simulink model "cmult_core"  (R2013a)
settings: Solver=ode45  StartTime=0.0  StopTime=10.0  RelTol=1e-3
libraries: xbsIndex_r4 x2035, casper_library_misc x116, casper_library_multipliers x36
(part 3 of 23)

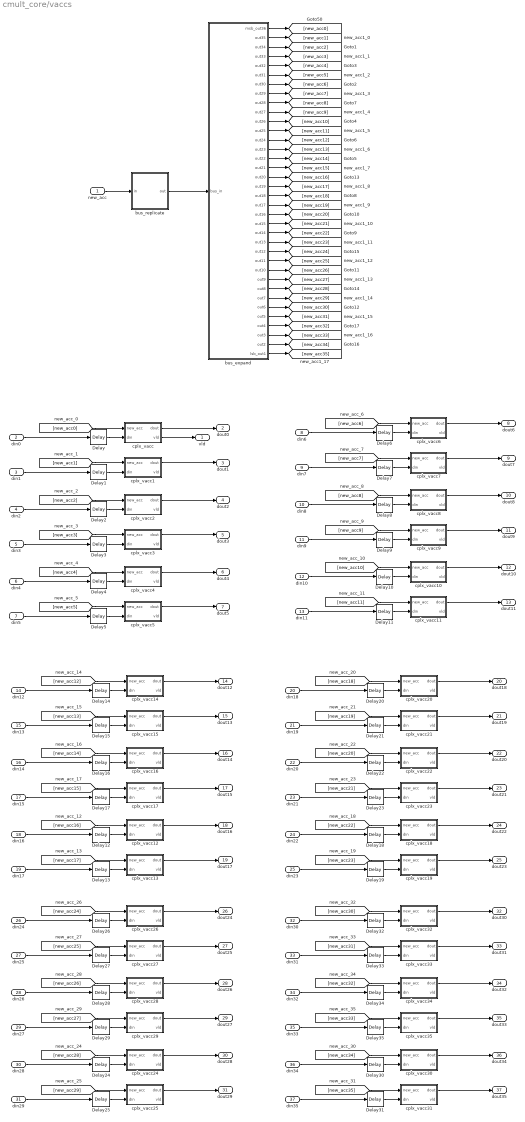
== system cmult_core/vaccs ==
  new_acc : Inport
  din0 : Inport  Port=2
  din1 : Inport  Port=3
  din2 : Inport  Port=4
  din3 : Inport  Port=5
  din4 : Inport  Port=6
  din5 : Inport  Port=7
  din6 : Inport  Port=8
  din7 : Inport  Port=9
  din8 : Inport  Port=10
  din9 : Inport  Port=11
  din10 : Inport  Port=12
  din11 : Inport  Port=13
  din12 : Inport  Port=14
  din13 : Inport  Port=15
  din14 : Inport  Port=16
  din15 : Inport  Port=17
  din16 : Inport  Port=18
  din17 : Inport  Port=19
  din18 : Inport  Port=20
  din19 : Inport  Port=21
  din20 : Inport  Port=22
  din21 : Inport  Port=23
  din22 : Inport  Port=24
  din23 : Inport  Port=25
  din24 : Inport  Port=26
  din25 : Inport  Port=27
  din26 : Inport  Port=28
  din27 : Inport  Port=29
  din28 : Inport  Port=30
  din29 : Inport  Port=31
  din30 : Inport  Port=32
  din31 : Inport  Port=33
  din32 : Inport  Port=34
  din33 : Inport  Port=35
  din34 : Inport  Port=36
  din35 : Inport  Port=37
  Delay{,1..35} (36 alike) : xbsIndex_r4/Delay  rst=off  infoeditControl=Selection of Reset will increase slice count due to use of real FFs and instead of SRLs  en=off  latency=5  dbl_ovrd=off  reg_retiming=on  block_type=delay
  bus_expand : Subsystem  AncestorBlock=casper_library_flow_control/bus_expand  mask(bus_expand){mode=divisions of equal size, outputNum=36, outputWidth=1, outputBinaryPt=0, outputArithmeticType=2, show_format=off, outputToWorkspace=off, variablePrefix=out, outputToModelAsWell=on}
      mask prompts: outputNum "Number of outputs:"; outputWidth "Output width:"; outputBinaryPt "Output binary point position:"; outputArithmeticType "Output arithmetic type (ufix=0, fix=1, bool=2):"; show_format "Print format string?"; outputToWorkspace "Output to workspace?"; variablePrefix "Variable name prefix:"; outputToModelAsWell "Output to model as well?"
      mask help:
      | Expands a 'bus' made using a bus_create or Xilinx
      | concat block.
      | The input will be divided into the specified number
      | of outputs with the specified arithmetic types.
      | Divisions are made from most significant bit.
      mask init: same as cmult_core/cross_multiplier/unpack0
      settings: AttributesFormatString=36 outputs
      mask TypeOptions mode: divisions of equal size | divisions of arbitrary size
      mask Callback mode: bus_expand_callback();
      mask Callback outputWidth: bus_expand_callback();
      mask Callback outputToWorkspace: bus_expand_callback();
  bus_replicate : Subsystem  AncestorBlock=casper_library_bus/bus_replicate  mask(bus_replicate){replication=36, latency=5, misc=off, implementation=core}
      mask prompts: replication "replication factor"; misc "misc support"; implementation "delay implementation"
      mask help: Output bus formed by replicating input bus a number of times
      mask init:
      | bus_replicate_init(gcb, ...
      |     'replication', replication, ...
      |     'latency', latency, ...
      |     'implementation', implementation, ...
      |     'misc', misc);
      mask TypeOptions implementation: core | behavioral
  cplx_vacc : Subsystem  mask{vacc_len=vacc_len}
      mask prompts: vacc_len "vector length"
  cplx_vacc1 : Subsystem  mask{vacc_len=vacc_len}
      mask prompts: vacc_len "vector length"
  cplx_vacc10 : Subsystem  mask{vacc_len=vacc_len}
      mask prompts: vacc_len "vector length"
  cplx_vacc11 : Subsystem  mask{vacc_len=vacc_len}
      mask prompts: vacc_len "vector length"
  cplx_vacc12 : Subsystem  mask{vacc_len=vacc_len}
      mask prompts: vacc_len "vector length"
  cplx_vacc13 : Subsystem  mask{vacc_len=vacc_len}
      mask prompts: vacc_len "vector length"
  cplx_vacc14 : Subsystem  mask{vacc_len=vacc_len}
      mask prompts: vacc_len "vector length"
  cplx_vacc15 : Subsystem  mask{vacc_len=vacc_len}
      mask prompts: vacc_len "vector length"
  cplx_vacc16 : Subsystem  mask{vacc_len=vacc_len}
      mask prompts: vacc_len "vector length"
  cplx_vacc17 : Subsystem  mask{vacc_len=vacc_len}
      mask prompts: vacc_len "vector length"
  cplx_vacc18 : Subsystem  mask{vacc_len=vacc_len}
      mask prompts: vacc_len "vector length"
  cplx_vacc19 : Subsystem  mask{vacc_len=vacc_len}
      mask prompts: vacc_len "vector length"
  cplx_vacc2 : Subsystem  mask{vacc_len=vacc_len}
      mask prompts: vacc_len "vector length"
  cplx_vacc20 : Subsystem  mask{vacc_len=vacc_len}
      mask prompts: vacc_len "vector length"
  cplx_vacc21 : Subsystem  mask{vacc_len=vacc_len}
      mask prompts: vacc_len "vector length"
  cplx_vacc22 : Subsystem  mask{vacc_len=vacc_len}
      mask prompts: vacc_len "vector length"
  cplx_vacc23 : Subsystem  mask{vacc_len=vacc_len}
      mask prompts: vacc_len "vector length"
  cplx_vacc24 : Subsystem  mask{vacc_len=vacc_len}
      mask prompts: vacc_len "vector length"
  cplx_vacc25 : Subsystem  mask{vacc_len=vacc_len}
      mask prompts: vacc_len "vector length"
  cplx_vacc26 : Subsystem  mask{vacc_len=vacc_len}
      mask prompts: vacc_len "vector length"
  cplx_vacc27 : Subsystem  mask{vacc_len=vacc_len}
      mask prompts: vacc_len "vector length"
  cplx_vacc28 : Subsystem  mask{vacc_len=vacc_len}
      mask prompts: vacc_len "vector length"
  cplx_vacc29 : Subsystem  mask{vacc_len=vacc_len}
      mask prompts: vacc_len "vector length"
  cplx_vacc3 : Subsystem  mask{vacc_len=vacc_len}
      mask prompts: vacc_len "vector length"
  cplx_vacc30 : Subsystem  mask{vacc_len=vacc_len}
      mask prompts: vacc_len "vector length"
  cplx_vacc31 : Subsystem  mask{vacc_len=vacc_len}
      mask prompts: vacc_len "vector length"
  cplx_vacc32 : Subsystem  mask{vacc_len=vacc_len}
      mask prompts: vacc_len "vector length"
  cplx_vacc33 : Subsystem  mask{vacc_len=vacc_len}
      mask prompts: vacc_len "vector length"
  cplx_vacc34 : Subsystem  mask{vacc_len=vacc_len}
      mask prompts: vacc_len "vector length"
  cplx_vacc35 : Subsystem  mask{vacc_len=vacc_len}
      mask prompts: vacc_len "vector length"
  cplx_vacc4 : Subsystem  mask{vacc_len=vacc_len}
      mask prompts: vacc_len "vector length"
  cplx_vacc5 : Subsystem  mask{vacc_len=vacc_len}
      mask prompts: vacc_len "vector length"
  cplx_vacc6 : Subsystem  mask{vacc_len=vacc_len}
      mask prompts: vacc_len "vector length"
  cplx_vacc7 : Subsystem  mask{vacc_len=vacc_len}
      mask prompts: vacc_len "vector length"
  cplx_vacc8 : Subsystem  mask{vacc_len=vacc_len}
      mask prompts: vacc_len "vector length"
  cplx_vacc9 : Subsystem  mask{vacc_len=vacc_len}
      mask prompts: vacc_len "vector length"
  vld : Outport
  dout0 : Outport  Port=2
  dout1 : Outport  Port=3
  dout2 : Outport  Port=4
  dout3 : Outport  Port=5
  dout4 : Outport  Port=6
  dout5 : Outport  Port=7
  dout6 : Outport  Port=8
  dout7 : Outport  Port=9
  dout8 : Outport  Port=10
  dout9 : Outport  Port=11
  dout10 : Outport  Port=12
  dout11 : Outport  Port=13
  dout12 : Outport  Port=14
  dout13 : Outport  Port=15
  dout14 : Outport  Port=16
  dout15 : Outport  Port=17
  dout16 : Outport  Port=18
  dout17 : Outport  Port=19
  dout18 : Outport  Port=20
  dout19 : Outport  Port=21
  dout20 : Outport  Port=22
  dout21 : Outport  Port=23
  dout22 : Outport  Port=24
  dout23 : Outport  Port=25
  dout24 : Outport  Port=26
  dout25 : Outport  Port=27
  dout26 : Outport  Port=28
  dout27 : Outport  Port=29
  dout28 : Outport  Port=30
  dout29 : Outport  Port=31
  dout30 : Outport  Port=32
  dout31 : Outport  Port=33
  dout32 : Outport  Port=34
  dout33 : Outport  Port=35
  dout34 : Outport  Port=36
  dout35 : Outport  Port=37
  wires:
  cplx_vacc/1(dout) -> dout0/1
  cplx_vacc/2(vld) -> vld/1
  din0/1 -> Delay/1
  [new_acc0] -> cplx_vacc/1(new_acc)
  new_acc/1 -> bus_replicate/1(in)
  bus_replicate/1(out) -> bus_expand/1(bus_in)
  bus_expand/28(out9) -> [new_acc27]
  bus_expand/36(lsb_out1) -> [new_acc35]
  bus_expand/35(out2) -> [new_acc34]
  bus_expand/30(out7) -> [new_acc29]
  bus_expand/23(out14) -> [new_acc22]
  bus_expand/24(out13) -> [new_acc23]
  bus_expand/32(out5) -> [new_acc31]
  bus_expand/11(out26) -> [new_acc10]
  bus_expand/31(out6) -> [new_acc30]
  bus_expand/15(out22) -> [new_acc14]
  bus_expand/8(out29) -> [new_acc7]
  bus_expand/26(out11) -> [new_acc25]
  bus_expand/33(out4) -> [new_acc32]
  bus_expand/22(out15) -> [new_acc21]
  bus_expand/34(out3) -> [new_acc33]
  bus_expand/27(out10) -> [new_acc26]
  bus_expand/9(out28) -> [new_acc8]
  bus_expand/18(out19) -> [new_acc17]
  bus_expand/6(out31) -> [new_acc5]
  bus_expand/10(out27) -> [new_acc9]
  bus_expand/13(out24) -> [new_acc12]
  bus_expand/25(out12) -> [new_acc24]
  bus_expand/14(out23) -> [new_acc13]
  bus_expand/20(out17) -> [new_acc19]
  bus_expand/19(out18) -> [new_acc18]
  bus_expand/3(out34) -> [new_acc2]
  bus_expand/29(out8) -> [new_acc28]
  bus_expand/7(out30) -> [new_acc6]
  bus_expand/16(out21) -> [new_acc15]
  bus_expand/4(out33) -> [new_acc3]
  bus_expand/1(msb_out36) -> [new_acc0]
  bus_expand/2(out35) -> [new_acc1]
  bus_expand/17(out20) -> [new_acc16]
  bus_expand/21(out16) -> [new_acc20]
  bus_expand/12(out25) -> [new_acc11]
  bus_expand/5(out32) -> [new_acc4]
  Delay/1 -> cplx_vacc/2(din)
  cplx_vacc1/1(dout) -> dout1/1
  din1/1 -> Delay1/1
  [new_acc1] -> cplx_vacc1/1(new_acc)
  Delay1/1 -> cplx_vacc1/2(din)
  cplx_vacc2/1(dout) -> dout2/1
  din2/1 -> Delay2/1
  [new_acc2] -> cplx_vacc2/1(new_acc)
  Delay2/1 -> cplx_vacc2/2(din)
  cplx_vacc3/1(dout) -> dout3/1
  din3/1 -> Delay3/1
  [new_acc3] -> cplx_vacc3/1(new_acc)
  Delay3/1 -> cplx_vacc3/2(din)
  cplx_vacc4/1(dout) -> dout4/1
  din4/1 -> Delay4/1
  [new_acc4] -> cplx_vacc4/1(new_acc)
  Delay4/1 -> cplx_vacc4/2(din)
  cplx_vacc5/1(dout) -> dout5/1
  din5/1 -> Delay5/1
  [new_acc5] -> cplx_vacc5/1(new_acc)
  Delay5/1 -> cplx_vacc5/2(din)
  cplx_vacc6/1(dout) -> dout6/1
  din6/1 -> Delay6/1
  [new_acc6] -> cplx_vacc6/1(new_acc)
  Delay6/1 -> cplx_vacc6/2(din)
  cplx_vacc7/1(dout) -> dout7/1
  din7/1 -> Delay7/1
  [new_acc7] -> cplx_vacc7/1(new_acc)
  Delay7/1 -> cplx_vacc7/2(din)
  cplx_vacc8/1(dout) -> dout8/1
  din8/1 -> Delay8/1
  [new_acc8] -> cplx_vacc8/1(new_acc)
  Delay8/1 -> cplx_vacc8/2(din)
  cplx_vacc9/1(dout) -> dout9/1
  din9/1 -> Delay9/1
  [new_acc9] -> cplx_vacc9/1(new_acc)
  Delay9/1 -> cplx_vacc9/2(din)
  cplx_vacc10/1(dout) -> dout10/1
  din10/1 -> Delay10/1
  [new_acc10] -> cplx_vacc10/1(new_acc)
  Delay10/1 -> cplx_vacc10/2(din)
  cplx_vacc11/1(dout) -> dout11/1
  din11/1 -> Delay11/1
  [new_acc11] -> cplx_vacc11/1(new_acc)
  Delay11/1 -> cplx_vacc11/2(din)
  cplx_vacc14/1(dout) -> dout12/1
  din12/1 -> Delay14/1
  [new_acc12] -> cplx_vacc14/1(new_acc)
  Delay14/1 -> cplx_vacc14/2(din)
  cplx_vacc15/1(dout) -> dout13/1
  din13/1 -> Delay15/1
  [new_acc13] -> cplx_vacc15/1(new_acc)
  Delay15/1 -> cplx_vacc15/2(din)
  cplx_vacc16/1(dout) -> dout14/1
  din14/1 -> Delay16/1
  [new_acc14] -> cplx_vacc16/1(new_acc)
  Delay16/1 -> cplx_vacc16/2(din)
  cplx_vacc17/1(dout) -> dout15/1
  din15/1 -> Delay17/1
  [new_acc15] -> cplx_vacc17/1(new_acc)
  Delay17/1 -> cplx_vacc17/2(din)
  cplx_vacc12/1(dout) -> dout16/1
  din16/1 -> Delay12/1
  [new_acc16] -> cplx_vacc12/1(new_acc)
  Delay12/1 -> cplx_vacc12/2(din)
  cplx_vacc13/1(dout) -> dout17/1
  din17/1 -> Delay13/1
  [new_acc17] -> cplx_vacc13/1(new_acc)
  Delay13/1 -> cplx_vacc13/2(din)
  cplx_vacc20/1(dout) -> dout18/1
  din18/1 -> Delay20/1
  [new_acc18] -> cplx_vacc20/1(new_acc)
  Delay20/1 -> cplx_vacc20/2(din)
  cplx_vacc21/1(dout) -> dout19/1
  din19/1 -> Delay21/1
  [new_acc19] -> cplx_vacc21/1(new_acc)
  Delay21/1 -> cplx_vacc21/2(din)
  cplx_vacc22/1(dout) -> dout20/1
  din20/1 -> Delay22/1
  [new_acc20] -> cplx_vacc22/1(new_acc)
  Delay22/1 -> cplx_vacc22/2(din)
  cplx_vacc23/1(dout) -> dout21/1
  din21/1 -> Delay23/1
  [new_acc21] -> cplx_vacc23/1(new_acc)
  Delay23/1 -> cplx_vacc23/2(din)
  cplx_vacc18/1(dout) -> dout22/1
  din22/1 -> Delay18/1
  [new_acc22] -> cplx_vacc18/1(new_acc)
  Delay18/1 -> cplx_vacc18/2(din)
  cplx_vacc19/1(dout) -> dout23/1
  din23/1 -> Delay19/1
  [new_acc23] -> cplx_vacc19/1(new_acc)
  Delay19/1 -> cplx_vacc19/2(din)
  cplx_vacc26/1(dout) -> dout24/1
  din24/1 -> Delay26/1
  [new_acc24] -> cplx_vacc26/1(new_acc)
  Delay26/1 -> cplx_vacc26/2(din)
  cplx_vacc27/1(dout) -> dout25/1
  din25/1 -> Delay27/1
  [new_acc25] -> cplx_vacc27/1(new_acc)
  Delay27/1 -> cplx_vacc27/2(din)
  cplx_vacc28/1(dout) -> dout26/1
  din26/1 -> Delay28/1
  [new_acc26] -> cplx_vacc28/1(new_acc)
  Delay28/1 -> cplx_vacc28/2(din)
  cplx_vacc29/1(dout) -> dout27/1
  din27/1 -> Delay29/1
  [new_acc27] -> cplx_vacc29/1(new_acc)
  Delay29/1 -> cplx_vacc29/2(din)
  cplx_vacc24/1(dout) -> dout28/1
  din28/1 -> Delay24/1
  [new_acc28] -> cplx_vacc24/1(new_acc)
  Delay24/1 -> cplx_vacc24/2(din)
  cplx_vacc25/1(dout) -> dout29/1
  din29/1 -> Delay25/1
  [new_acc29] -> cplx_vacc25/1(new_acc)
  Delay25/1 -> cplx_vacc25/2(din)
  cplx_vacc32/1(dout) -> dout30/1
  din30/1 -> Delay32/1
  [new_acc30] -> cplx_vacc32/1(new_acc)
  Delay32/1 -> cplx_vacc32/2(din)
  cplx_vacc33/1(dout) -> dout31/1
  din31/1 -> Delay33/1
  [new_acc31] -> cplx_vacc33/1(new_acc)
  Delay33/1 -> cplx_vacc33/2(din)
  cplx_vacc34/1(dout) -> dout32/1
  din32/1 -> Delay34/1
  [new_acc32] -> cplx_vacc34/1(new_acc)
  Delay34/1 -> cplx_vacc34/2(din)
  cplx_vacc35/1(dout) -> dout33/1
  din33/1 -> Delay35/1
  [new_acc33] -> cplx_vacc35/1(new_acc)
  Delay35/1 -> cplx_vacc35/2(din)
  cplx_vacc30/1(dout) -> dout34/1
  din34/1 -> Delay30/1
  [new_acc34] -> cplx_vacc30/1(new_acc)
  Delay30/1 -> cplx_vacc30/2(din)
  cplx_vacc31/1(dout) -> dout35/1
  din35/1 -> Delay31/1
  [new_acc35] -> cplx_vacc31/1(new_acc)
  Delay31/1 -> cplx_vacc31/2(din)

== system cmult_core/cross_multiplier/cvrt0_0_0_imag ==
  din : Inport
  convert : Subsystem  AncestorBlock=casper_library_misc/convert  mask(convert){bin_pt_in=binary_point_i, n_bits_out=bit_width_o, bin_pt_out=binary_point_o, quantization=Truncate, overflow=Wrap, latency=latency, adder_imp=Fabric}
      mask prompts: bin_pt_in "Binary Point In"; n_bits_out "Bit Width Out"; bin_pt_out "Binary Point Out"; adder_imp "Adder Implementation"
      mask help:
      | Convert input value to the specified bit width and precision.
      |
      | Does not support upscaling number of fractional bits (eg 8_5 to 8_4 is ok, but not 8_4 to 8_5).
      mask init:
      | convert_init(gcb, ...
      |     'bin_pt_in',bin_pt_in, ...
      |     'n_bits_out',n_bits_out,...
      |     'bin_pt_out',bin_pt_out, ...
      |     'quantization',quantization,...
      |     'overflow',overflow,...
      |     'latency',latency,...
      |     'adder_imp',adder_imp);
      settings: AttributesFormatString=|
      | N_14 ==> 17_14
      | truncate, wrap
      | latency = 0
      mask Help:
      | <pre>
      | Description::
      | 
      | Outputs converted version of the input.
      | 
      | Mask Parameters::
      | 
      | Binary Point In (bin_pt_in): Specifies the binary point location in the input.
      | 
      | Bit Width Out (n_bits_out): Specifies the width of the output.
      | 
      | Binary Point Out (bin_pt_out): Specifies the binary point location in the output.
      | 
      | Quantization (quantization): Specifies quantization handling.
      | 
      | Overflow (overflow): Specifies overflow handling.
      | 
      | Latency (latency): Specifies the latency of the underlying adder block, which is the overall
      | latency of this block as well.
      | Adder Implementation (adder_imp) specifies whether the adder should be implemented in DSP or logic. In either case, pipelining is enabled.</pre>
      mask TypeOptions quantization: Truncate | Round  (unbiased: +/- Inf) | Round  (unbiased: Even Values) | Round  (unbiased: Zero) | Round  (unbiased: Odd Values) | Round  (biased: Up) | Round  (biased: Down)
      mask TypeOptions overflow: Wrap | Saturate | Error
      mask TypeOptions adder_imp: Fabric | DSP48 | Behavioural
  never : xbsIndex_r4/Constant  const=0  gui_display_data_type=Fixed-point  arith_type=Boolean  n_bits=16  bin_pt=14  preci_type=Single  exp_width=8  frac_width=24  explicit_period=on  period=1  equ=P=C  opselect=C  inp2=PCIN>>17  opr=+  inp1=P  carry=CIN  dbl_ovrd=off  block_type=constant
  dout : Outport
  of : Outport  Port=2
  wires:
  din/1 -> convert/1(in)
  convert/1(out) -> dout/1
  never/1 -> of/1

== system cmult_core/cross_multiplier/cvrt0_0_0_real ==
  din : Inport
  convert : Subsystem  AncestorBlock=casper_library_misc/convert  mask(convert){bin_pt_in=binary_point_i, n_bits_out=bit_width_o, bin_pt_out=binary_point_o, quantization=Truncate, overflow=Wrap, latency=latency, adder_imp=Fabric}
      mask prompts: bin_pt_in "Binary Point In"; n_bits_out "Bit Width Out"; bin_pt_out "Binary Point Out"; adder_imp "Adder Implementation"
      mask help:
      | Convert input value to the specified bit width and precision.
      |
      | Does not support upscaling number of fractional bits (eg 8_5 to 8_4 is ok, but not 8_4 to 8_5).
      mask init: same as cmult_core/cross_multiplier/cvrt0_0_0_imag/convert
      settings: AttributesFormatString=|
      | N_14 ==> 17_14
      | truncate, wrap
      | latency = 0
      mask Help:
      | <pre>
      | Description::
      | 
      | Outputs converted version of the input.
      | 
      | Mask Parameters::
      | 
      | Binary Point In (bin_pt_in): Specifies the binary point location in the input.
      | 
      | Bit Width Out (n_bits_out): Specifies the width of the output.
      | 
      | Binary Point Out (bin_pt_out): Specifies the binary point location in the output.
      | 
      | Quantization (quantization): Specifies quantization handling.
      | 
      | Overflow (overflow): Specifies overflow handling.
      | 
      | Latency (latency): Specifies the latency of the underlying adder block, which is the overall
      | latency of this block as well.
      | Adder Implementation (adder_imp) specifies whether the adder should be implemented in DSP or logic. In either case, pipelining is enabled.</pre>
      mask TypeOptions quantization: Truncate | Round  (unbiased: +/- Inf) | Round  (unbiased: Even Values) | Round  (unbiased: Zero) | Round  (unbiased: Odd Values) | Round  (biased: Up) | Round  (biased: Down)
      mask TypeOptions overflow: Wrap | Saturate | Error
      mask TypeOptions adder_imp: Fabric | DSP48 | Behavioural
  never : xbsIndex_r4/Constant  const=0  gui_display_data_type=Fixed-point  arith_type=Boolean  n_bits=16  bin_pt=14  preci_type=Single  exp_width=8  frac_width=24  explicit_period=on  period=1  equ=P=C  opselect=C  inp2=PCIN>>17  opr=+  inp1=P  carry=CIN  dbl_ovrd=off  block_type=constant
  dout : Outport
  of : Outport  Port=2
  wires:
  din/1 -> convert/1(in)
  convert/1(out) -> dout/1
  never/1 -> of/1

== system cmult_core/cross_multiplier/cvrt0_1_0_imag ==
  din : Inport
  convert : Subsystem  AncestorBlock=casper_library_misc/convert  mask(convert){bin_pt_in=binary_point_i, n_bits_out=bit_width_o, bin_pt_out=binary_point_o, quantization=Truncate, overflow=Wrap, latency=latency, adder_imp=Fabric}
      mask prompts: bin_pt_in "Binary Point In"; n_bits_out "Bit Width Out"; bin_pt_out "Binary Point Out"; adder_imp "Adder Implementation"
      mask help:
      | Convert input value to the specified bit width and precision.
      |
      | Does not support upscaling number of fractional bits (eg 8_5 to 8_4 is ok, but not 8_4 to 8_5).
      mask init: same as cmult_core/cross_multiplier/cvrt0_0_0_imag/convert
      settings: AttributesFormatString=|
      | N_14 ==> 17_14
      | truncate, wrap
      | latency = 0
      mask Help:
      | <pre>
      | Description::
      | 
      | Outputs converted version of the input.
      | 
      | Mask Parameters::
      | 
      | Binary Point In (bin_pt_in): Specifies the binary point location in the input.
      | 
      | Bit Width Out (n_bits_out): Specifies the width of the output.
      | 
      | Binary Point Out (bin_pt_out): Specifies the binary point location in the output.
      | 
      | Quantization (quantization): Specifies quantization handling.
      | 
      | Overflow (overflow): Specifies overflow handling.
      | 
      | Latency (latency): Specifies the latency of the underlying adder block, which is the overall
      | latency of this block as well.
      | Adder Implementation (adder_imp) specifies whether the adder should be implemented in DSP or logic. In either case, pipelining is enabled.</pre>
      mask TypeOptions quantization: Truncate | Round  (unbiased: +/- Inf) | Round  (unbiased: Even Values) | Round  (unbiased: Zero) | Round  (unbiased: Odd Values) | Round  (biased: Up) | Round  (biased: Down)
      mask TypeOptions overflow: Wrap | Saturate | Error
      mask TypeOptions adder_imp: Fabric | DSP48 | Behavioural
  never : xbsIndex_r4/Constant  const=0  gui_display_data_type=Fixed-point  arith_type=Boolean  n_bits=16  bin_pt=14  preci_type=Single  exp_width=8  frac_width=24  explicit_period=on  period=1  equ=P=C  opselect=C  inp2=PCIN>>17  opr=+  inp1=P  carry=CIN  dbl_ovrd=off  block_type=constant
  dout : Outport
  of : Outport  Port=2
  wires:
  din/1 -> convert/1(in)
  convert/1(out) -> dout/1
  never/1 -> of/1

== system cmult_core/cross_multiplier/cvrt0_1_0_real ==
  din : Inport
  convert : Subsystem  AncestorBlock=casper_library_misc/convert  mask(convert){bin_pt_in=binary_point_i, n_bits_out=bit_width_o, bin_pt_out=binary_point_o, quantization=Truncate, overflow=Wrap, latency=latency, adder_imp=Fabric}
      mask prompts: bin_pt_in "Binary Point In"; n_bits_out "Bit Width Out"; bin_pt_out "Binary Point Out"; adder_imp "Adder Implementation"
      mask help:
      | Convert input value to the specified bit width and precision.
      |
      | Does not support upscaling number of fractional bits (eg 8_5 to 8_4 is ok, but not 8_4 to 8_5).
      mask init: same as cmult_core/cross_multiplier/cvrt0_0_0_imag/convert
      settings: AttributesFormatString=|
      | N_14 ==> 17_14
      | truncate, wrap
      | latency = 0
      mask Help:
      | <pre>
      | Description::
      | 
      | Outputs converted version of the input.
      | 
      | Mask Parameters::
      | 
      | Binary Point In (bin_pt_in): Specifies the binary point location in the input.
      | 
      | Bit Width Out (n_bits_out): Specifies the width of the output.
      | 
      | Binary Point Out (bin_pt_out): Specifies the binary point location in the output.
      | 
      | Quantization (quantization): Specifies quantization handling.
      | 
      | Overflow (overflow): Specifies overflow handling.
      | 
      | Latency (latency): Specifies the latency of the underlying adder block, which is the overall
      | latency of this block as well.
      | Adder Implementation (adder_imp) specifies whether the adder should be implemented in DSP or logic. In either case, pipelining is enabled.</pre>
      mask TypeOptions quantization: Truncate | Round  (unbiased: +/- Inf) | Round  (unbiased: Even Values) | Round  (unbiased: Zero) | Round  (unbiased: Odd Values) | Round  (biased: Up) | Round  (biased: Down)
      mask TypeOptions overflow: Wrap | Saturate | Error
      mask TypeOptions adder_imp: Fabric | DSP48 | Behavioural
  never : xbsIndex_r4/Constant  const=0  gui_display_data_type=Fixed-point  arith_type=Boolean  n_bits=16  bin_pt=14  preci_type=Single  exp_width=8  frac_width=24  explicit_period=on  period=1  equ=P=C  opselect=C  inp2=PCIN>>17  opr=+  inp1=P  carry=CIN  dbl_ovrd=off  block_type=constant
  dout : Outport
  of : Outport  Port=2
  wires:
  din/1 -> convert/1(in)
  convert/1(out) -> dout/1
  never/1 -> of/1

== system cmult_core/cross_multiplier/cvrt0_2_0_imag ==
  din : Inport
  convert : Subsystem  AncestorBlock=casper_library_misc/convert  mask(convert){bin_pt_in=binary_point_i, n_bits_out=bit_width_o, bin_pt_out=binary_point_o, quantization=Truncate, overflow=Wrap, latency=latency, adder_imp=Fabric}
      mask prompts: bin_pt_in "Binary Point In"; n_bits_out "Bit Width Out"; bin_pt_out "Binary Point Out"; adder_imp "Adder Implementation"
      mask help:
      | Convert input value to the specified bit width and precision.
      |
      | Does not support upscaling number of fractional bits (eg 8_5 to 8_4 is ok, but not 8_4 to 8_5).
      mask init: same as cmult_core/cross_multiplier/cvrt0_0_0_imag/convert
      settings: AttributesFormatString=|
      | N_14 ==> 17_14
      | truncate, wrap
      | latency = 0
      mask Help:
      | <pre>
      | Description::
      | 
      | Outputs converted version of the input.
      | 
      | Mask Parameters::
      | 
      | Binary Point In (bin_pt_in): Specifies the binary point location in the input.
      | 
      | Bit Width Out (n_bits_out): Specifies the width of the output.
      | 
      | Binary Point Out (bin_pt_out): Specifies the binary point location in the output.
      | 
      | Quantization (quantization): Specifies quantization handling.
      | 
      | Overflow (overflow): Specifies overflow handling.
      | 
      | Latency (latency): Specifies the latency of the underlying adder block, which is the overall
      | latency of this block as well.
      | Adder Implementation (adder_imp) specifies whether the adder should be implemented in DSP or logic. In either case, pipelining is enabled.</pre>
      mask TypeOptions quantization: Truncate | Round  (unbiased: +/- Inf) | Round  (unbiased: Even Values) | Round  (unbiased: Zero) | Round  (unbiased: Odd Values) | Round  (biased: Up) | Round  (biased: Down)
      mask TypeOptions overflow: Wrap | Saturate | Error
      mask TypeOptions adder_imp: Fabric | DSP48 | Behavioural
  never : xbsIndex_r4/Constant  const=0  gui_display_data_type=Fixed-point  arith_type=Boolean  n_bits=16  bin_pt=14  preci_type=Single  exp_width=8  frac_width=24  explicit_period=on  period=1  equ=P=C  opselect=C  inp2=PCIN>>17  opr=+  inp1=P  carry=CIN  dbl_ovrd=off  block_type=constant
  dout : Outport
  of : Outport  Port=2
  wires:
  din/1 -> convert/1(in)
  convert/1(out) -> dout/1
  never/1 -> of/1

== system cmult_core/cross_multiplier/cvrt0_2_0_real ==
  din : Inport
  convert : Subsystem  AncestorBlock=casper_library_misc/convert  mask(convert){bin_pt_in=binary_point_i, n_bits_out=bit_width_o, bin_pt_out=binary_point_o, quantization=Truncate, overflow=Wrap, latency=latency, adder_imp=Fabric}
      mask prompts: bin_pt_in "Binary Point In"; n_bits_out "Bit Width Out"; bin_pt_out "Binary Point Out"; adder_imp "Adder Implementation"
      mask help:
      | Convert input value to the specified bit width and precision.
      |
      | Does not support upscaling number of fractional bits (eg 8_5 to 8_4 is ok, but not 8_4 to 8_5).
      mask init: same as cmult_core/cross_multiplier/cvrt0_0_0_imag/convert
      settings: AttributesFormatString=|
      | N_14 ==> 17_14
      | truncate, wrap
      | latency = 0
      mask Help:
      | <pre>
      | Description::
      | 
      | Outputs converted version of the input.
      | 
      | Mask Parameters::
      | 
      | Binary Point In (bin_pt_in): Specifies the binary point location in the input.
      | 
      | Bit Width Out (n_bits_out): Specifies the width of the output.
      | 
      | Binary Point Out (bin_pt_out): Specifies the binary point location in the output.
      | 
      | Quantization (quantization): Specifies quantization handling.
      | 
      | Overflow (overflow): Specifies overflow handling.
      | 
      | Latency (latency): Specifies the latency of the underlying adder block, which is the overall
      | latency of this block as well.
      | Adder Implementation (adder_imp) specifies whether the adder should be implemented in DSP or logic. In either case, pipelining is enabled.</pre>
      mask TypeOptions quantization: Truncate | Round  (unbiased: +/- Inf) | Round  (unbiased: Even Values) | Round  (unbiased: Zero) | Round  (unbiased: Odd Values) | Round  (biased: Up) | Round  (biased: Down)
      mask TypeOptions overflow: Wrap | Saturate | Error
      mask TypeOptions adder_imp: Fabric | DSP48 | Behavioural
  never : xbsIndex_r4/Constant  const=0  gui_display_data_type=Fixed-point  arith_type=Boolean  n_bits=16  bin_pt=14  preci_type=Single  exp_width=8  frac_width=24  explicit_period=on  period=1  equ=P=C  opselect=C  inp2=PCIN>>17  opr=+  inp1=P  carry=CIN  dbl_ovrd=off  block_type=constant
  dout : Outport
  of : Outport  Port=2
  wires:
  din/1 -> convert/1(in)
  convert/1(out) -> dout/1
  never/1 -> of/1

== system cmult_core/cross_multiplier/cvrt0_3_0_imag ==
  din : Inport
  convert : Subsystem  AncestorBlock=casper_library_misc/convert  mask(convert){bin_pt_in=binary_point_i, n_bits_out=bit_width_o, bin_pt_out=binary_point_o, quantization=Truncate, overflow=Wrap, latency=latency, adder_imp=Fabric}
      mask prompts: bin_pt_in "Binary Point In"; n_bits_out "Bit Width Out"; bin_pt_out "Binary Point Out"; adder_imp "Adder Implementation"
      mask help:
      | Convert input value to the specified bit width and precision.
      |
      | Does not support upscaling number of fractional bits (eg 8_5 to 8_4 is ok, but not 8_4 to 8_5).
      mask init: same as cmult_core/cross_multiplier/cvrt0_0_0_imag/convert
      settings: AttributesFormatString=|
      | N_14 ==> 17_14
      | truncate, wrap
      | latency = 0
      mask Help:
      | <pre>
      | Description::
      | 
      | Outputs converted version of the input.
      | 
      | Mask Parameters::
      | 
      | Binary Point In (bin_pt_in): Specifies the binary point location in the input.
      | 
      | Bit Width Out (n_bits_out): Specifies the width of the output.
      | 
      | Binary Point Out (bin_pt_out): Specifies the binary point location in the output.
      | 
      | Quantization (quantization): Specifies quantization handling.
      | 
      | Overflow (overflow): Specifies overflow handling.
      | 
      | Latency (latency): Specifies the latency of the underlying adder block, which is the overall
      | latency of this block as well.
      | Adder Implementation (adder_imp) specifies whether the adder should be implemented in DSP or logic. In either case, pipelining is enabled.</pre>
      mask TypeOptions quantization: Truncate | Round  (unbiased: +/- Inf) | Round  (unbiased: Even Values) | Round  (unbiased: Zero) | Round  (unbiased: Odd Values) | Round  (biased: Up) | Round  (biased: Down)
      mask TypeOptions overflow: Wrap | Saturate | Error
      mask TypeOptions adder_imp: Fabric | DSP48 | Behavioural
  never : xbsIndex_r4/Constant  const=0  gui_display_data_type=Fixed-point  arith_type=Boolean  n_bits=16  bin_pt=14  preci_type=Single  exp_width=8  frac_width=24  explicit_period=on  period=1  equ=P=C  opselect=C  inp2=PCIN>>17  opr=+  inp1=P  carry=CIN  dbl_ovrd=off  block_type=constant
  dout : Outport
  of : Outport  Port=2
  wires:
  din/1 -> convert/1(in)
  convert/1(out) -> dout/1
  never/1 -> of/1

== system cmult_core/cross_multiplier/cvrt0_3_0_real ==
  din : Inport
  convert : Subsystem  AncestorBlock=casper_library_misc/convert  mask(convert){bin_pt_in=binary_point_i, n_bits_out=bit_width_o, bin_pt_out=binary_point_o, quantization=Truncate, overflow=Wrap, latency=latency, adder_imp=Fabric}
      mask prompts: bin_pt_in "Binary Point In"; n_bits_out "Bit Width Out"; bin_pt_out "Binary Point Out"; adder_imp "Adder Implementation"
      mask help:
      | Convert input value to the specified bit width and precision.
      |
      | Does not support upscaling number of fractional bits (eg 8_5 to 8_4 is ok, but not 8_4 to 8_5).
      mask init: same as cmult_core/cross_multiplier/cvrt0_0_0_imag/convert
      settings: AttributesFormatString=|
      | N_14 ==> 17_14
      | truncate, wrap
      | latency = 0
      mask Help:
      | <pre>
      | Description::
      | 
      | Outputs converted version of the input.
      | 
      | Mask Parameters::
      | 
      | Binary Point In (bin_pt_in): Specifies the binary point location in the input.
      | 
      | Bit Width Out (n_bits_out): Specifies the width of the output.
      | 
      | Binary Point Out (bin_pt_out): Specifies the binary point location in the output.
      | 
      | Quantization (quantization): Specifies quantization handling.
      | 
      | Overflow (overflow): Specifies overflow handling.
      | 
      | Latency (latency): Specifies the latency of the underlying adder block, which is the overall
      | latency of this block as well.
      | Adder Implementation (adder_imp) specifies whether the adder should be implemented in DSP or logic. In either case, pipelining is enabled.</pre>
      mask TypeOptions quantization: Truncate | Round  (unbiased: +/- Inf) | Round  (unbiased: Even Values) | Round  (unbiased: Zero) | Round  (unbiased: Odd Values) | Round  (biased: Up) | Round  (biased: Down)
      mask TypeOptions overflow: Wrap | Saturate | Error
      mask TypeOptions adder_imp: Fabric | DSP48 | Behavioural
  never : xbsIndex_r4/Constant  const=0  gui_display_data_type=Fixed-point  arith_type=Boolean  n_bits=16  bin_pt=14  preci_type=Single  exp_width=8  frac_width=24  explicit_period=on  period=1  equ=P=C  opselect=C  inp2=PCIN>>17  opr=+  inp1=P  carry=CIN  dbl_ovrd=off  block_type=constant
  dout : Outport
  of : Outport  Port=2
  wires:
  din/1 -> convert/1(in)
  convert/1(out) -> dout/1
  never/1 -> of/1

== system cmult_core/cross_multiplier/cvrt0_4_0_imag ==
  din : Inport
  convert : Subsystem  AncestorBlock=casper_library_misc/convert  mask(convert){bin_pt_in=binary_point_i, n_bits_out=bit_width_o, bin_pt_out=binary_point_o, quantization=Truncate, overflow=Wrap, latency=latency, adder_imp=Fabric}
      mask prompts: bin_pt_in "Binary Point In"; n_bits_out "Bit Width Out"; bin_pt_out "Binary Point Out"; adder_imp "Adder Implementation"
      mask help:
      | Convert input value to the specified bit width and precision.
      |
      | Does not support upscaling number of fractional bits (eg 8_5 to 8_4 is ok, but not 8_4 to 8_5).
      mask init: same as cmult_core/cross_multiplier/cvrt0_0_0_imag/convert
      settings: AttributesFormatString=|
      | N_14 ==> 17_14
      | truncate, wrap
      | latency = 0
      mask Help:
      | <pre>
      | Description::
      | 
      | Outputs converted version of the input.
      | 
      | Mask Parameters::
      | 
      | Binary Point In (bin_pt_in): Specifies the binary point location in the input.
      | 
      | Bit Width Out (n_bits_out): Specifies the width of the output.
      | 
      | Binary Point Out (bin_pt_out): Specifies the binary point location in the output.
      | 
      | Quantization (quantization): Specifies quantization handling.
      | 
      | Overflow (overflow): Specifies overflow handling.
      | 
      | Latency (latency): Specifies the latency of the underlying adder block, which is the overall
      | latency of this block as well.
      | Adder Implementation (adder_imp) specifies whether the adder should be implemented in DSP or logic. In either case, pipelining is enabled.</pre>
      mask TypeOptions quantization: Truncate | Round  (unbiased: +/- Inf) | Round  (unbiased: Even Values) | Round  (unbiased: Zero) | Round  (unbiased: Odd Values) | Round  (biased: Up) | Round  (biased: Down)
      mask TypeOptions overflow: Wrap | Saturate | Error
      mask TypeOptions adder_imp: Fabric | DSP48 | Behavioural
  never : xbsIndex_r4/Constant  const=0  gui_display_data_type=Fixed-point  arith_type=Boolean  n_bits=16  bin_pt=14  preci_type=Single  exp_width=8  frac_width=24  explicit_period=on  period=1  equ=P=C  opselect=C  inp2=PCIN>>17  opr=+  inp1=P  carry=CIN  dbl_ovrd=off  block_type=constant
  dout : Outport
  of : Outport  Port=2
  wires:
  din/1 -> convert/1(in)
  convert/1(out) -> dout/1
  never/1 -> of/1

== system cmult_core/cross_multiplier/cvrt0_4_0_real ==
  din : Inport
  convert : Subsystem  AncestorBlock=casper_library_misc/convert  mask(convert){bin_pt_in=binary_point_i, n_bits_out=bit_width_o, bin_pt_out=binary_point_o, quantization=Truncate, overflow=Wrap, latency=latency, adder_imp=Fabric}
      mask prompts: bin_pt_in "Binary Point In"; n_bits_out "Bit Width Out"; bin_pt_out "Binary Point Out"; adder_imp "Adder Implementation"
      mask help:
      | Convert input value to the specified bit width and precision.
      |
      | Does not support upscaling number of fractional bits (eg 8_5 to 8_4 is ok, but not 8_4 to 8_5).
      mask init: same as cmult_core/cross_multiplier/cvrt0_0_0_imag/convert
      settings: AttributesFormatString=|
      | N_14 ==> 17_14
      | truncate, wrap
      | latency = 0
      mask Help:
      | <pre>
      | Description::
      | 
      | Outputs converted version of the input.
      | 
      | Mask Parameters::
      | 
      | Binary Point In (bin_pt_in): Specifies the binary point location in the input.
      | 
      | Bit Width Out (n_bits_out): Specifies the width of the output.
      | 
      | Binary Point Out (bin_pt_out): Specifies the binary point location in the output.
      | 
      | Quantization (quantization): Specifies quantization handling.
      | 
      | Overflow (overflow): Specifies overflow handling.
      | 
      | Latency (latency): Specifies the latency of the underlying adder block, which is the overall
      | latency of this block as well.
      | Adder Implementation (adder_imp) specifies whether the adder should be implemented in DSP or logic. In either case, pipelining is enabled.</pre>
      mask TypeOptions quantization: Truncate | Round  (unbiased: +/- Inf) | Round  (unbiased: Even Values) | Round  (unbiased: Zero) | Round  (unbiased: Odd Values) | Round  (biased: Up) | Round  (biased: Down)
      mask TypeOptions overflow: Wrap | Saturate | Error
      mask TypeOptions adder_imp: Fabric | DSP48 | Behavioural
  never : xbsIndex_r4/Constant  const=0  gui_display_data_type=Fixed-point  arith_type=Boolean  n_bits=16  bin_pt=14  preci_type=Single  exp_width=8  frac_width=24  explicit_period=on  period=1  equ=P=C  opselect=C  inp2=PCIN>>17  opr=+  inp1=P  carry=CIN  dbl_ovrd=off  block_type=constant
  dout : Outport
  of : Outport  Port=2
  wires:
  din/1 -> convert/1(in)
  convert/1(out) -> dout/1
  never/1 -> of/1

== system cmult_core/cross_multiplier/cvrt0_5_0_imag ==
  din : Inport
  convert : Subsystem  AncestorBlock=casper_library_misc/convert  mask(convert){bin_pt_in=binary_point_i, n_bits_out=bit_width_o, bin_pt_out=binary_point_o, quantization=Truncate, overflow=Wrap, latency=latency, adder_imp=Fabric}
      mask prompts: bin_pt_in "Binary Point In"; n_bits_out "Bit Width Out"; bin_pt_out "Binary Point Out"; adder_imp "Adder Implementation"
      mask help:
      | Convert input value to the specified bit width and precision.
      |
      | Does not support upscaling number of fractional bits (eg 8_5 to 8_4 is ok, but not 8_4 to 8_5).
      mask init: same as cmult_core/cross_multiplier/cvrt0_0_0_imag/convert
      settings: AttributesFormatString=|
      | N_14 ==> 17_14
      | truncate, wrap
      | latency = 0
      mask Help:
      | <pre>
      | Description::
      | 
      | Outputs converted version of the input.
      | 
      | Mask Parameters::
      | 
      | Binary Point In (bin_pt_in): Specifies the binary point location in the input.
      | 
      | Bit Width Out (n_bits_out): Specifies the width of the output.
      | 
      | Binary Point Out (bin_pt_out): Specifies the binary point location in the output.
      | 
      | Quantization (quantization): Specifies quantization handling.
      | 
      | Overflow (overflow): Specifies overflow handling.
      | 
      | Latency (latency): Specifies the latency of the underlying adder block, which is the overall
      | latency of this block as well.
      | Adder Implementation (adder_imp) specifies whether the adder should be implemented in DSP or logic. In either case, pipelining is enabled.</pre>
      mask TypeOptions quantization: Truncate | Round  (unbiased: +/- Inf) | Round  (unbiased: Even Values) | Round  (unbiased: Zero) | Round  (unbiased: Odd Values) | Round  (biased: Up) | Round  (biased: Down)
      mask TypeOptions overflow: Wrap | Saturate | Error
      mask TypeOptions adder_imp: Fabric | DSP48 | Behavioural
  never : xbsIndex_r4/Constant  const=0  gui_display_data_type=Fixed-point  arith_type=Boolean  n_bits=16  bin_pt=14  preci_type=Single  exp_width=8  frac_width=24  explicit_period=on  period=1  equ=P=C  opselect=C  inp2=PCIN>>17  opr=+  inp1=P  carry=CIN  dbl_ovrd=off  block_type=constant
  dout : Outport
  of : Outport  Port=2
  wires:
  din/1 -> convert/1(in)
  convert/1(out) -> dout/1
  never/1 -> of/1

== system cmult_core/cross_multiplier/cvrt0_5_0_real ==
  din : Inport
  convert : Subsystem  AncestorBlock=casper_library_misc/convert  mask(convert){bin_pt_in=binary_point_i, n_bits_out=bit_width_o, bin_pt_out=binary_point_o, quantization=Truncate, overflow=Wrap, latency=latency, adder_imp=Fabric}
      mask prompts: bin_pt_in "Binary Point In"; n_bits_out "Bit Width Out"; bin_pt_out "Binary Point Out"; adder_imp "Adder Implementation"
      mask help:
      | Convert input value to the specified bit width and precision.
      |
      | Does not support upscaling number of fractional bits (eg 8_5 to 8_4 is ok, but not 8_4 to 8_5).
      mask init: same as cmult_core/cross_multiplier/cvrt0_0_0_imag/convert
      settings: AttributesFormatString=|
      | N_14 ==> 17_14
      | truncate, wrap
      | latency = 0
      mask Help:
      | <pre>
      | Description::
      | 
      | Outputs converted version of the input.
      | 
      | Mask Parameters::
      | 
      | Binary Point In (bin_pt_in): Specifies the binary point location in the input.
      | 
      | Bit Width Out (n_bits_out): Specifies the width of the output.
      | 
      | Binary Point Out (bin_pt_out): Specifies the binary point location in the output.
      | 
      | Quantization (quantization): Specifies quantization handling.
      | 
      | Overflow (overflow): Specifies overflow handling.
      | 
      | Latency (latency): Specifies the latency of the underlying adder block, which is the overall
      | latency of this block as well.
      | Adder Implementation (adder_imp) specifies whether the adder should be implemented in DSP or logic. In either case, pipelining is enabled.</pre>
      mask TypeOptions quantization: Truncate | Round  (unbiased: +/- Inf) | Round  (unbiased: Even Values) | Round  (unbiased: Zero) | Round  (unbiased: Odd Values) | Round  (biased: Up) | Round  (biased: Down)
      mask TypeOptions overflow: Wrap | Saturate | Error
      mask TypeOptions adder_imp: Fabric | DSP48 | Behavioural
  never : xbsIndex_r4/Constant  const=0  gui_display_data_type=Fixed-point  arith_type=Boolean  n_bits=16  bin_pt=14  preci_type=Single  exp_width=8  frac_width=24  explicit_period=on  period=1  equ=P=C  opselect=C  inp2=PCIN>>17  opr=+  inp1=P  carry=CIN  dbl_ovrd=off  block_type=constant
  dout : Outport
  of : Outport  Port=2
  wires:
  din/1 -> convert/1(in)
  convert/1(out) -> dout/1
  never/1 -> of/1

== system cmult_core/cross_multiplier/cvrt0_6_0_imag ==
  din : Inport
  convert : Subsystem  AncestorBlock=casper_library_misc/convert  mask(convert){bin_pt_in=binary_point_i, n_bits_out=bit_width_o, bin_pt_out=binary_point_o, quantization=Truncate, overflow=Wrap, latency=latency, adder_imp=Fabric}
      mask prompts: bin_pt_in "Binary Point In"; n_bits_out "Bit Width Out"; bin_pt_out "Binary Point Out"; adder_imp "Adder Implementation"
      mask help:
      | Convert input value to the specified bit width and precision.
      |
      | Does not support upscaling number of fractional bits (eg 8_5 to 8_4 is ok, but not 8_4 to 8_5).
      mask init: same as cmult_core/cross_multiplier/cvrt0_0_0_imag/convert
      settings: AttributesFormatString=|
      | N_14 ==> 17_14
      | truncate, wrap
      | latency = 0
      mask Help:
      | <pre>
      | Description::
      | 
      | Outputs converted version of the input.
      | 
      | Mask Parameters::
      | 
      | Binary Point In (bin_pt_in): Specifies the binary point location in the input.
      | 
      | Bit Width Out (n_bits_out): Specifies the width of the output.
      | 
      | Binary Point Out (bin_pt_out): Specifies the binary point location in the output.
      | 
      | Quantization (quantization): Specifies quantization handling.
      | 
      | Overflow (overflow): Specifies overflow handling.
      | 
      | Latency (latency): Specifies the latency of the underlying adder block, which is the overall
      | latency of this block as well.
      | Adder Implementation (adder_imp) specifies whether the adder should be implemented in DSP or logic. In either case, pipelining is enabled.</pre>
      mask TypeOptions quantization: Truncate | Round  (unbiased: +/- Inf) | Round  (unbiased: Even Values) | Round  (unbiased: Zero) | Round  (unbiased: Odd Values) | Round  (biased: Up) | Round  (biased: Down)
      mask TypeOptions overflow: Wrap | Saturate | Error
      mask TypeOptions adder_imp: Fabric | DSP48 | Behavioural
  never : xbsIndex_r4/Constant  const=0  gui_display_data_type=Fixed-point  arith_type=Boolean  n_bits=16  bin_pt=14  preci_type=Single  exp_width=8  frac_width=24  explicit_period=on  period=1  equ=P=C  opselect=C  inp2=PCIN>>17  opr=+  inp1=P  carry=CIN  dbl_ovrd=off  block_type=constant
  dout : Outport
  of : Outport  Port=2
  wires:
  din/1 -> convert/1(in)
  convert/1(out) -> dout/1
  never/1 -> of/1

== system cmult_core/cross_multiplier/cvrt0_6_0_real ==
  din : Inport
  convert : Subsystem  AncestorBlock=casper_library_misc/convert  mask(convert){bin_pt_in=binary_point_i, n_bits_out=bit_width_o, bin_pt_out=binary_point_o, quantization=Truncate, overflow=Wrap, latency=latency, adder_imp=Fabric}
      mask prompts: bin_pt_in "Binary Point In"; n_bits_out "Bit Width Out"; bin_pt_out "Binary Point Out"; adder_imp "Adder Implementation"
      mask help:
      | Convert input value to the specified bit width and precision.
      |
      | Does not support upscaling number of fractional bits (eg 8_5 to 8_4 is ok, but not 8_4 to 8_5).
      mask init: same as cmult_core/cross_multiplier/cvrt0_0_0_imag/convert
      settings: AttributesFormatString=|
      | N_14 ==> 17_14
      | truncate, wrap
      | latency = 0
      mask Help:
      | <pre>
      | Description::
      | 
      | Outputs converted version of the input.
      | 
      | Mask Parameters::
      | 
      | Binary Point In (bin_pt_in): Specifies the binary point location in the input.
      | 
      | Bit Width Out (n_bits_out): Specifies the width of the output.
      | 
      | Binary Point Out (bin_pt_out): Specifies the binary point location in the output.
      | 
      | Quantization (quantization): Specifies quantization handling.
      | 
      | Overflow (overflow): Specifies overflow handling.
      | 
      | Latency (latency): Specifies the latency of the underlying adder block, which is the overall
      | latency of this block as well.
      | Adder Implementation (adder_imp) specifies whether the adder should be implemented in DSP or logic. In either case, pipelining is enabled.</pre>
      mask TypeOptions quantization: Truncate | Round  (unbiased: +/- Inf) | Round  (unbiased: Even Values) | Round  (unbiased: Zero) | Round  (unbiased: Odd Values) | Round  (biased: Up) | Round  (biased: Down)
      mask TypeOptions overflow: Wrap | Saturate | Error
      mask TypeOptions adder_imp: Fabric | DSP48 | Behavioural
  never : xbsIndex_r4/Constant  const=0  gui_display_data_type=Fixed-point  arith_type=Boolean  n_bits=16  bin_pt=14  preci_type=Single  exp_width=8  frac_width=24  explicit_period=on  period=1  equ=P=C  opselect=C  inp2=PCIN>>17  opr=+  inp1=P  carry=CIN  dbl_ovrd=off  block_type=constant
  dout : Outport
  of : Outport  Port=2
  wires:
  din/1 -> convert/1(in)
  convert/1(out) -> dout/1
  never/1 -> of/1
